simulink model "FOC_Motor_Control"  (R2020b)
settings: Solver=FixedStepAuto  StartTime=0.0  StopTime=10.0  FixedStep=Fixed_Step_Size  RelTol=1e-3
values from neighbouring files (symbols this model uses):
  atan_table = -1.5690511 -1.5690503 -1.5690495 -1.5690485 -1.5690477 -1.5690469 -1.569046 -1.5690452 -1.5690442 -1.5690434 -1.5690426 -1.5690417 -1.5690409 -1.5690399 -1.5690391 -1.5690383 -1.5690374 -1.5690365 -1.5690356 -1.5690348 -1.5690339 -1.569033 -1.5690322 -1.5690314 -1.5690304 -1.5690296 -1.5690287 -1.5690278 -1.5690269 -1.5690261 -1.5690252 -1.5690243 -1.5690234 -1.5690225 -1.5690217 -1.5690207 -1.569    [Motor_Control_Data.sldd]
  Cosine_table = 1.0 0.99999529 0.99999058 0.99998587 0.99998116 0.99996704 0.99995291 0.99993885 0.99992472 0.99990118 0.99987763 0.99985409 0.9998306 0.99979764 0.99976468 0.99973178 0.99969882 0.99965644 0.99961412 0.99957174 0.99952942 0.99947762 0.99942589 0.99937415 0.99932235 0.9992612 0.99920005 0.99913889 0.99907768 0.99900717 0.99893659 0.99886602 0.99879545 0.99871546 0.99863547 0.99855554 0.99847555 0.    [Motor_Control_Data.sldd]
  Dead_Com_Enable = 1.0    [Motor_Control_Data.sldd]
  Dead_Time = 2.5E-6    [Motor_Control_Data.sldd]
  Flux = 0.1125    [Motor_Control_Data.sldd]
  ID_Ki = 48.0    [Motor_Control_Data.sldd]
  ID_Kp = 0.84    [Motor_Control_Data.sldd]
  IQ_Ki = 48.0    [Motor_Control_Data.sldd]
  IQ_Kp = 1.869    [Motor_Control_Data.sldd]
  Ld = 0.00014    [Motor_Control_Data.sldd]
  Lq = 0.0003115    [Motor_Control_Data.sldd]
  Pole_Pairs = 4.0    [Motor_Control_Data.sldd]
  PWM_Frequency = 10000.0    [Motor_Control_Data.sldd]
  Sine_table = 0.0 0.0015339879 0.0030679768 0.0046019657 0.0061359555 0.0076698866 0.0092038177 0.010737749 0.012271681 0.013805497 0.015339312 0.016873131 0.018406944 0.019940587 0.021474229 0.023007872 0.024541514 0.026074925 0.027608337 0.029141748 0.03067516 0.032208283 0.033741407 0.035274528 0.036807653 0.038340431 0.039873205 0.04140598 0.042938754 0.04447113 0.046003502 0.047535874 0.049068246 0.0506001    [Motor_Control_Data.sldd]
  Speed_Ki = 10.809    [Motor_Control_Data.sldd]
  Speed_Kp = 0.08    [Motor_Control_Data.sldd]
  Speed_PI_OutputMax = 700.0    [Motor_Control_Data.sldd]
  Speed_PI_OutputMin = -700.0    [Motor_Control_Data.sldd]
  SpeedFilter_Fn = 0.2    [Motor_Control_Data.sldd]
  TorqueMode = 0.0    [Motor_Control_Data.sldd]
undefined symbols (not defined in the file or in its folder): DiscIntNeverNeededParam, inverter, LADRC_b0, LADRC_Omega_c, SVPWM
libraries: simulink x6
(part 1 of 2)
settings Model: DataDictionary=Motor_Control_Data.sldd  Creator=Administrator  LastModifiedBy=Administrator
settings OptimizationCC: DefaultParameterBehavior=Inlined  UseDivisionForNetSlopeComputation=on  GainParamInheritBuiltInType=on  UseFloatMulNetSlope=on  InlineInvariantSignals=on  PassReuseOutputArgsAs=Individual arguments  ZeroExternalMemoryAtStartup=off  ZeroInternalMemoryAtStartup=off  NoFixptDivByZeroProtection=on  EfficientFloat2IntCast=on  LifeSpan=1  OptimizeBlockOrder=speed  DifferentSizesBufferReuse=on  EfficientTunableParamExpr=on
settings DebuggingCC: ParameterTunabilityLossMsg=error
settings HardwareCC: ProdBitPerPointer=32  ProdBitPerSizeT=32  ProdBitPerPtrDiffT=32  ProdLargestAtomicInteger=Long  ProdLargestAtomicFloat=Double  ProdEndianess=BigEndian  ProdWordSize=32  ProdLongLongMode=on  ProdHWDeviceType=Freescale->32-bit PowerPC
settings ModelReferenceCC: ModelReferenceNumInstancesAllowed=Single
settings SFSimCC: MATLABDynamicMemAlloc=off
settings RTWCC: Description=Embedded Coder  SystemTargetFile=ert.tlc  GenCodeOnly=on  TemplateMakefile=ert_default_tmf  GenerateReport=on  BuildConfiguration=Faster Runs  LaunchReport=on
settings CodeAppCC: ForceParamTrailComments=on  IgnoreCustomStorageClasses=off  OperatorAnnotations=on  SimulinkDataObjDesc=on  SFDataObjDesc=on  CustomSymbolStrGlobalVar=rt$N$M  CustomSymbolStrType=$N$M  CustomSymbolStrFcn=$N$M$F  CustomSymbolStrMacro=$N$M  InsertBlockDesc=on
settings ERTTargetCC: TargetLangStandard=C99 (ISO)  GenerateSampleERTMain=on  IncludeMdlTerminateFcn=off  CombineSignalStateStructs=on  SupportComplex=off  SupportNonInlinedSFcns=on  InlinedParameterPlacement=NonHierarchical  ERTCustomFileTemplate=example_file_process.tlc

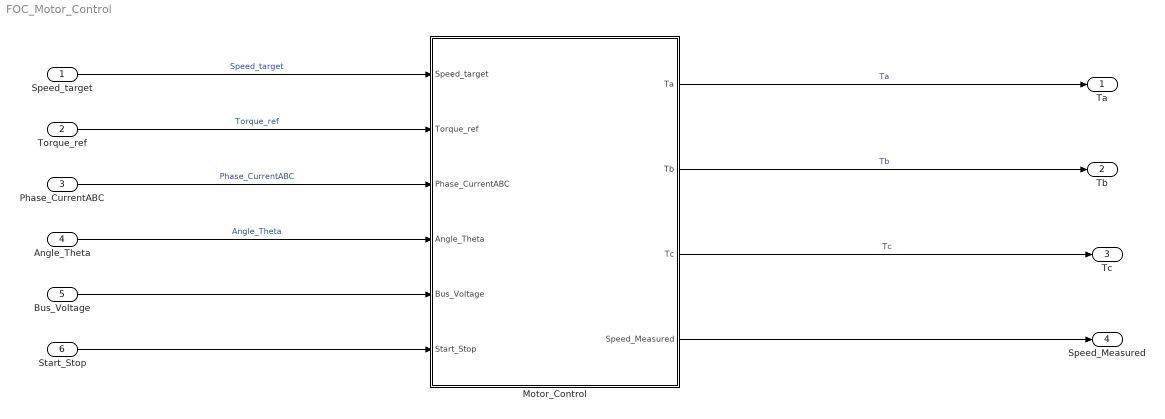
== system FOC_Motor_Control ==
  Speed_target : Inport
  Torque_ref : Inport  Port=2  OutMin=0  OutMax=2*pi  OutDataTypeStr=single
  Phase_CurrentABC : Inport  Port=3  OutDataTypeStr=single  PortDimensions=3
  Angle_Theta : Inport  Port=4  OutMin=0  OutMax=2*pi
  Bus_Voltage : Inport  Port=5
  Start_Stop : Inport  Port=6
  Motor_Control : Subsystem  TreatAsAtomicUnit=on
  Ta : Outport
  Tb : Outport  Port=2
  Tc : Outport  Port=3
  Speed_Measured : Outport  Port=4
  wires:
  Speed_target/1 -> Motor_Control/1(Speed_target)  "Speed_target"
  Motor_Control/1(Ta) -> Ta/1  "Ta"
  Motor_Control/3(Tc) -> Tc/1  "Tc"
  Motor_Control/2(Tb) -> Tb/1  "Tb"
  Phase_CurrentABC/1 -> Motor_Control/3(Phase_CurrentABC)  "Phase_CurrentABC"
  Angle_Theta/1 -> Motor_Control/4(Angle_Theta)  "Angle_Theta"
  Torque_ref/1 -> Motor_Control/2(Torque_ref)  "Torque_ref"
  Bus_Voltage/1 -> Motor_Control/5(Bus_Voltage)
  Start_Stop/1 -> Motor_Control/6(Start_Stop)
  Motor_Control/4(Speed_Measured) -> Speed_Measured/1

== system FOC_Motor_Control/Motor_Control ==
  Speed_target : Inport
  Torque_ref : Inport  Port=2  OutMin=0  OutMax=2*pi
  Phase_CurrentABC : Inport  Port=3  PortDimensions=3
  Angle_Theta : Inport  Port=4  OutMin=0  OutMax=2*pi
  Bus_Voltage : Inport  Port=5
  Start_Stop : Inport  Port=6
  Motor_Control_Function : Subsystem
  Ta : Outport
  Tb : Outport  Port=2
  Tc : Outport  Port=3
  Speed_Measured : Outport  Port=4
  wires:
  Motor_Control_Function/2(Tb) -> Tb/1
  Motor_Control_Function/3(Tc) -> Tc/1
  Motor_Control_Function/1(Ta) -> Ta/1
  Speed_target/1 -> Motor_Control_Function/1(Speed_target)  "Speed_target"
  Phase_CurrentABC/1 -> Motor_Control_Function/2(Phase_CurrentABC)  "Phase_CurrentABC"
  Angle_Theta/1 -> Motor_Control_Function/3(Angle_Theta)  "Angle_Theta"
  Start_Stop/1 -> Motor_Control_Function/5(Start_Stop)
  Bus_Voltage/1 -> Motor_Control_Function/4(Bus_voltage)
  Torque_ref/1 -> Motor_Control_Function/6(Torque_ref)
  Motor_Control_Function/5(Speed_Measured) -> Speed_Measured/1

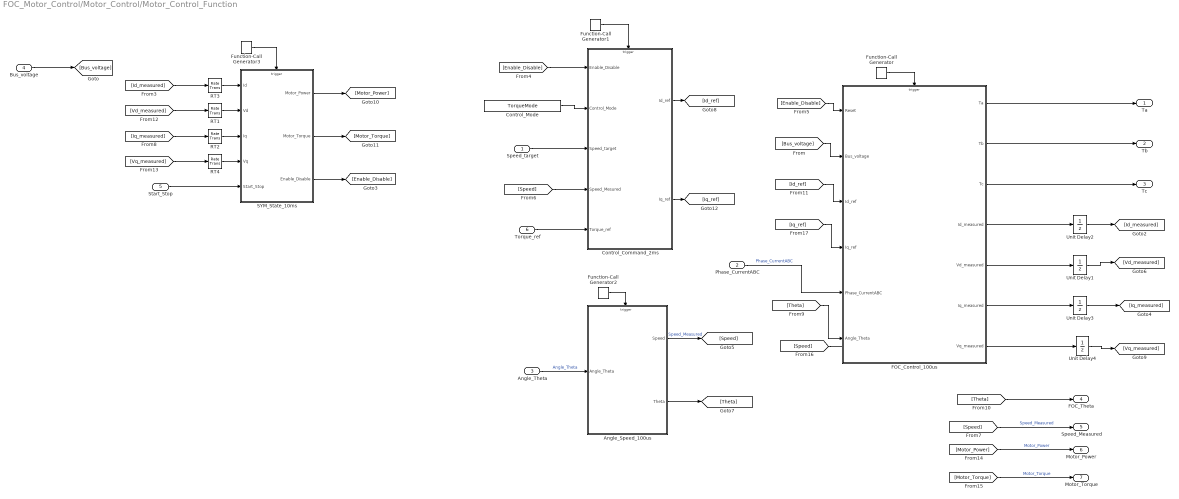
== system FOC_Motor_Control/Motor_Control/Motor_Control_Function ==
  Speed_target : Inport
  Phase_CurrentABC : Inport  Port=2  PortDimensions=3
  Angle_Theta : Inport  Port=3  OutMin=0  OutMax=2*pi
  Bus_voltage : Inport  Port=4
  Start_Stop : Inport  Port=5
  Torque_ref : Inport  Port=6  OutMin=0  OutMax=2*pi
  Angle_Speed_100us : Subsystem
      settings: RTWSystemCode=Nonreusable function  RTWFcnNameOpts=Use subsystem name  RTWFileNameOpts=Use subsystem name
  Control_Command_2ms : Subsystem  TreatAsAtomicUnit=on
      settings: RTWSystemCode=Nonreusable function  RTWFcnNameOpts=Use subsystem name  RTWFileNameOpts=Use subsystem name  FunctionInterfaceSpec=Allow arguments (Optimized)
  Control_Mode : Constant  Value=TorqueMode
  FOC_Control_100us : Subsystem  TreatAsAtomicUnit=on
      settings: RTWSystemCode=Nonreusable function  RTWFcnNameOpts=Use subsystem name  RTWFileNameOpts=Use subsystem name  FunctionInterfaceSpec=Allow arguments (Optimized)
  Function-Call Generator : simulink/Ports & Subsystems/Function-Call Generator  sample_time=1/PWM_Frequency  numberOfIterations=1  DisallowWideOutput=off
  Function-Call Generator1 : simulink/Ports & Subsystems/Function-Call Generator  sample_time=Task_2ms  numberOfIterations=1  DisallowWideOutput=off
  Function-Call Generator2 : simulink/Ports & Subsystems/Function-Call Generator  sample_time=1/PWM_Frequency  numberOfIterations=1  DisallowWideOutput=off
  Function-Call Generator3 : simulink/Ports & Subsystems/Function-Call Generator  sample_time=Task_10ms  numberOfIterations=1  DisallowWideOutput=off
  RT{1..4} (4 alike) : RateTransition  Integrity=off
  SYM_State_10ms : Subsystem
      settings: RTWSystemCode=Nonreusable function  RTWFcnNameOpts=Use subsystem name  RTWFileNameOpts=Use subsystem name
  Unit Delay{1..4} (4 alike) : UnitDelay  SampleTime=-1  HasFrameUpgradeWarning=on
  Ta : Outport
  Tb : Outport  Port=2
  Tc : Outport  Port=3
  FOC_Theta : Outport  Port=4
  Speed_Measured : Outport  Port=5
  Motor_Power : Outport  Port=6
  Motor_Torque : Outport  Port=7
  wires:
  Function-Call Generator1/1 -> Control_Command_2ms/Trigger
  Control_Mode/1 -> Control_Command_2ms/2(Control_Mode)
  Angle_Theta/1 -> Angle_Speed_100us/1(Angle_Theta)  "Angle_Theta"
  Function-Call Generator/1 -> FOC_Control_100us/Trigger
  Phase_CurrentABC/1 -> FOC_Control_100us/5(Phase_CurrentABC)  "Phase_CurrentABC"
  FOC_Control_100us/3(Tc) -> Tc/1
  Speed_target/1 -> Control_Command_2ms/3(Speed_target)
  FOC_Control_100us/2(Tb) -> Tb/1
  FOC_Control_100us/1(Ta) -> Ta/1
  Function-Call Generator2/1 -> Angle_Speed_100us/Trigger
  Function-Call Generator3/1 -> SYM_State_10ms/Trigger
  SYM_State_10ms/3(Enable_Disable) -> [Enable_Disable]
  [Enable_Disable] -> Control_Command_2ms/1(Enable_Disable)
  [Enable_Disable] -> FOC_Control_100us/1(Reset)
  Angle_Speed_100us/1(Speed) -> [Speed]  "Speed_Measured"
  [Speed] -> Speed_Measured/1  "Speed_Measured"
  Angle_Speed_100us/2(Theta) -> [Theta]
  [Theta] -> FOC_Control_100us/6(Angle_Theta)
  [Theta] -> FOC_Theta/1
  Control_Command_2ms/1(Id_ref) -> [Id_ref]
  [Id_ref] -> FOC_Control_100us/3(Id_ref)
  Start_Stop/1 -> SYM_State_10ms/5(Start_Stop)
  Bus_voltage/1 -> [Bus_voltage]
  FOC_Control_100us/6(Iq_measured) -> Unit Delay3/1
  FOC_Control_100us/7(Vq_measured) -> Unit Delay4/1
  FOC_Control_100us/4(Id_measured) -> Unit Delay2/1
  FOC_Control_100us/5(Vd_measured) -> Unit Delay1/1
  Unit Delay2/1 -> [Id_measured]
  Unit Delay1/1 -> [Vd_measured]
  Unit Delay3/1 -> [Iq_measured]
  Unit Delay4/1 -> [Vq_measured]
  [Iq_measured] -> RT2/1
  [Id_measured] -> RT3/1
  [Vd_measured] -> RT1/1
  [Vq_measured] -> RT4/1
  SYM_State_10ms/1(Motor_Power) -> [Motor_Power]
  [Motor_Power] -> Motor_Power/1  "Motor_Power"
  RT3/1 -> SYM_State_10ms/1(Id)
  RT1/1 -> SYM_State_10ms/2(Vd)
  RT2/1 -> SYM_State_10ms/3(Iq)
  RT4/1 -> SYM_State_10ms/4(Vq)
  [Bus_voltage] -> FOC_Control_100us/2(Bus_voltage)
  SYM_State_10ms/2(Motor_Torque) -> [Motor_Torque]
  [Motor_Torque] -> Motor_Torque/1  "Motor_Torque"
  Torque_ref/1 -> Control_Command_2ms/5(Torque_ref)
  [Speed] -> ?
  [Speed] -> Control_Command_2ms/4(Speed_Mesured)
  Control_Command_2ms/2(Iq_ref) -> [Iq_ref]
  [Iq_ref] -> FOC_Control_100us/4(Iq_ref)

== system FOC_Motor_Control/Motor_Control/Motor_Control_Function/Angle_Speed_100us ==
  Angle_Theta : Inport  OutMin=0  OutMax=2*pi
  Trigger : TriggerPort  TriggerType=function-call  VariantControl=Variant  SampleTimeType=periodic  SampleTime=-1  PortDimensions=1
  Speed_Resolver : Subsystem  TreatAsAtomicUnit=on
      settings: RTWSystemCode=Nonreusable function  RTWFcnNameOpts=Use subsystem name
  Speed : Outport
  Theta : Outport  Port=2
  wires:
  Speed_Resolver/1(Speed_out) -> Speed/1
  Speed_Resolver/2(Dir_Angle) -> Theta/1
  Angle_Theta/1 -> Speed_Resolver/1(Theta)  "Angle_Theta"

== system FOC_Motor_Control/Motor_Control/Motor_Control_Function/Control_Command_2ms ==
  Enable_Disable : Inport
  Control_Mode : Inport  Port=2
  Speed_target : Inport  Port=3
  Speed_Mesured : Inport  Port=4  OutMin=0  OutMax=2*pi
  Torque_ref : Inport  Port=5  OutMin=0  OutMax=2*pi
  Trigger : TriggerPort  TriggerType=function-call  VariantControl=Variant  SampleTimeType=periodic  SampleTime=-1  PortDimensions=1
  Constant : Constant  Value=0  OutDataTypeStr=single
  Control_Command_2ms : Subsystem  TreatAsAtomicUnit=on
      settings: RTWSystemCode=Nonreusable function  RTWFcnNameOpts=Use subsystem name  RTWFileNameOpts=Use subsystem name  FunctionInterfaceSpec=Allow arguments (Optimized)
  Id_ref : Outport
  Iq_ref : Outport  Port=2
  wires:
  Control_Mode/1 -> Control_Command_2ms/2(Control_Mode)
  Speed_target/1 -> Control_Command_2ms/3(Speed_target)
  Speed_Mesured/1 -> Control_Command_2ms/4(Speed_Mesured)
  Enable_Disable/1 -> Control_Command_2ms/1(Reset)
  Torque_ref/1 -> Control_Command_2ms/5(Torque_ref)
  Control_Command_2ms/1(Te_ref) -> Iq_ref/1  "Iq_ref"
  Constant/1 -> Id_ref/1  "Id_ref"

== system FOC_Motor_Control/Motor_Control/Motor_Control_Function/FOC_Control_100us ==
  Reset : Inport
  Bus_voltage : Inport  Port=2
  Id_ref : Inport  Port=3
  Iq_ref : Inport  Port=4
  Phase_CurrentABC : Inport  Port=5  PortDimensions=3
  Angle_Theta : Inport  Port=6  OutMin=0  OutMax=2*pi
  Trigger : TriggerPort  TriggerType=function-call  VariantControl=Variant  SampleTimeType=periodic  SampleTime=-1  PortDimensions=1
  FOC : Subsystem  TreatAsAtomicUnit=on
      settings: RTWSystemCode=Nonreusable function  RTWFcnNameOpts=Use subsystem name
  Ta : Outport
  Tb : Outport  Port=2
  Tc : Outport  Port=3
  Id_measured : Outport  Port=4
  Vd_measured : Outport  Port=5
  Iq_measured : Outport  Port=6
  Vq_measured : Outport  Port=7
  wires:
  FOC/1(Ta) -> Ta/1  "Ta"
  FOC/2(Tb) -> Tb/1  "Tb"
  FOC/3(Tc) -> Tc/1  "Tc"
  Angle_Theta/1 -> FOC/5(Angle_Theta)  "Angle_Theta"
  Phase_CurrentABC/1 -> FOC/6(Phase_CurrentABC)  "Phase_CurrentABC"
  Reset/1 -> FOC/1(Reset)
  FOC/6(Iq_measured) -> Iq_measured/1
  FOC/7(Vq_measured) -> Vq_measured/1
  FOC/4(Id_measured) -> Id_measured/1
  FOC/5(Vd_measured) -> Vd_measured/1
  Bus_voltage/1 -> FOC/2(Bus_voltage)
  Id_ref/1 -> FOC/3(Id_target)  "Id_ref"
  Iq_ref/1 -> FOC/4(Iq_target)  "Iq_ref"

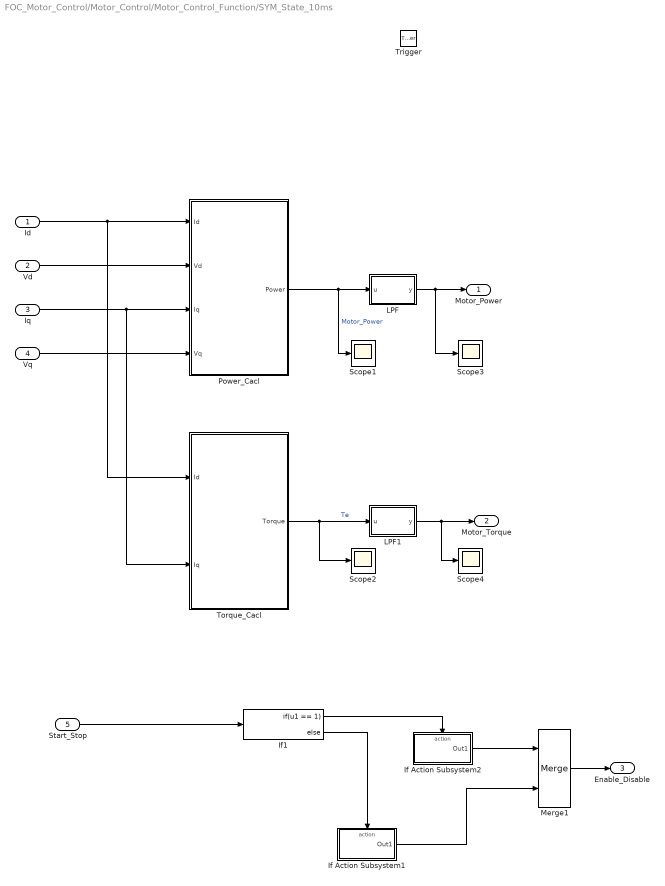
== system FOC_Motor_Control/Motor_Control/Motor_Control_Function/SYM_State_10ms ==
  Id : Inport
  Vd : Inport  Port=2
  Iq : Inport  Port=3
  Vq : Inport  Port=4
  Start_Stop : Inport  Port=5  OutDataTypeStr=uint8
  Trigger : TriggerPort  TriggerType=function-call  VariantControl=Variant  SampleTimeType=periodic  SampleTime=-1  PortDimensions=1
  If Action Subsystem1 : Subsystem  TreatAsAtomicUnit=on
  If Action Subsystem2 : Subsystem  TreatAsAtomicUnit=on
  If1 : If  IfExpression=u1 == 1
  LPF : Subsystem
  LPF1 : Subsystem
  Merge1 : Merge
  Power_Cacl : Subsystem
  Scope{1..4} (4 alike) : Scope
  Torque_Cacl : Subsystem
  Motor_Power : Outport
  Motor_Torque : Outport  Port=2
  Enable_Disable : Outport  Port=3
  wires:
  Iq/1 -> Torque_Cacl/2(Iq), Power_Cacl/3(Iq)
  Vq/1 -> Power_Cacl/4(Vq)
  Power_Cacl/1(Power) -> LPF/1(u), Scope1/1  "Motor_Power"
  Vd/1 -> Power_Cacl/2(Vd)
  Id/1 -> Torque_Cacl/1(Id), Power_Cacl/1(Id)
  LPF/1(y) -> Scope3/1, Motor_Power/1
  Torque_Cacl/1(Torque) -> LPF1/1(u), Scope2/1  "Te"
  LPF1/1(y) -> Motor_Torque/1, Scope4/1
  Start_Stop/1 -> If1/1
  If1/2 -> If Action Subsystem1/Action
  If1/1 -> If Action Subsystem2/Action
  If Action Subsystem2/1(Out1) -> Merge1/1
  If Action Subsystem1/1(Out1) -> Merge1/2
  Merge1/1 -> Enable_Disable/1

== system FOC_Motor_Control/Motor_Control/Motor_Control_Function/Angle_Speed_100us/Speed_Resolver ==
  Theta : Inport
  DT2 : DataTypeConversion  OutDataTypeStr=single
  Speed_cacl : Subsystem  TreatAsAtomicUnit=on
      settings: RTWSystemCode=Nonreusable function  RTWFcnNameOpts=Use subsystem name
  Speed_out : Outport
  Dir_Angle : Outport  Port=2
  wires:
  Theta/1 -> DT2/1, Speed_cacl/1(position)
  Speed_cacl/1(Speed_RPM) -> Speed_out/1  "Speed_Measured"
  DT2/1 -> Dir_Angle/1  "Direct_Angle"

== system FOC_Motor_Control/Motor_Control/Motor_Control_Function/Control_Command_2ms/Control_Command_2ms ==
  Reset : Inport
  Control_Mode : Inport  Port=2
  Speed_target : Inport  Port=3
  Speed_Mesured : Inport  Port=4  OutMin=0  OutMax=2*pi
  Torque_ref : Inport  Port=5  OutMin=0  OutMax=2*pi
  Merge : Merge
  Speed_PI : Subsystem  TreatAsAtomicUnit=on  SystemSampleTime=inverter.Ts
      settings: RTWSystemCode=Nonreusable function
  Switch Case : SwitchCase  CaseConditions={0,1}
  Switch Case Action Subsystem : Subsystem  TreatAsAtomicUnit=on
      settings: RTWSystemCode=Nonreusable function
  Te_ref : Outport
  wires:
  Switch Case Action Subsystem/1(Iq_out) -> Merge/2
  Torque_ref/1 -> Switch Case Action Subsystem/1(Iq_in)
  Switch Case/3 -> [default]
  [Torque_Mode] -> Switch Case Action Subsystem/Action
  Switch Case/2 -> [Torque_Mode]
  Switch Case/1 -> [Speed_Mode]
  Control_Mode/1 -> Switch Case/1
  [Speed_Mode] -> Speed_PI/Action
  Speed_PI/1(Iq_ref) -> Merge/1  "Iq_ref"
  Merge/1 -> Te_ref/1
  Speed_target/1 -> Speed_PI/1(Speed_Command)
  Reset/1 -> Speed_PI/3(Reset)
  Speed_Mesured/1 -> Speed_PI/2(Speed_Measured)

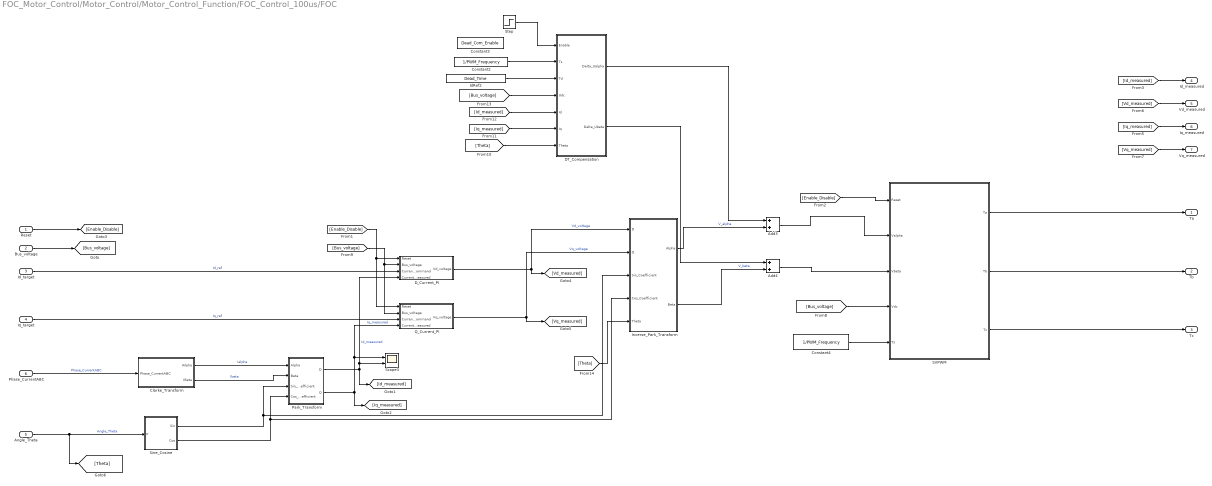
== system FOC_Motor_Control/Motor_Control/Motor_Control_Function/FOC_Control_100us/FOC ==
  Reset : Inport
  Bus_voltage : Inport  Port=2
  Id_target : Inport  Port=3
  Iq_target : Inport  Port=4
  Angle_Theta : Inport  Port=5  OutMin=0  OutMax=2*pi
  Phase_CurrentABC : Inport  Port=6  PortDimensions=3
  Add3 : Sum  OutDataTypeStr=single
  Add4 : Sum  OutDataTypeStr=single
  Clarke_Transform : Subsystem  TreatAsAtomicUnit=on
      settings: RTWSystemCode=Nonreusable function  RTWFcnNameOpts=Use subsystem name
  Constant2 : Constant  Value=1/PWM_Frequency  OutDataTypeStr=single
  Constant3 : Constant  Value=Dead_Com_Enable  OutDataTypeStr=single
  Constant4 : Constant  Value=1/PWM_Frequency  OutDataTypeStr=single
  DT_Compensation : Subsystem  TreatAsAtomicUnit=on
      settings: RTWSystemCode=Nonreusable function  RTWFcnNameOpts=Use subsystem name
  D_Current_PI : Subsystem  TreatAsAtomicUnit=on
      settings: RTWSystemCode=Nonreusable function  RTWFcnNameOpts=Use subsystem name
  IdRef2 : Constant  Value=Dead_Time  OutDataTypeStr=single
  Inverse_Park_Transform : Subsystem  TreatAsAtomicUnit=on
      settings: RTWSystemCode=Nonreusable function  RTWFcnNameOpts=Use subsystem name
      mask Display:
      | port_label('input',1,'D')
      | port_label('input',2,'Q')
      | port_label('input',3,'Sin')
      | port_label('input',4,'Cos')
      | port_label('output',1,'\alpha','texmode', 'on')
      | port_label('output',2,'\beta','texmode', 'on')
  Park_Transform : Subsystem  TreatAsAtomicUnit=on
      settings: RTWSystemCode=Nonreusable function  RTWFcnNameOpts=Use subsystem name
      mask Display:
      | port_label('input',1,'\alpha','texmode', 'on')
      | port_label('input',2,'\beta','texmode', 'on')
      | port_label('input',3,'Sin')
      | port_label('input',4,'Cos')
      | port_label('output',1,'D')
      | port_label('output',2,'Q')
  Q_Current_PI : Subsystem  TreatAsAtomicUnit=on
      settings: RTWSystemCode=Nonreusable function  RTWFcnNameOpts=Use subsystem name
  SVPWM : Subsystem  AncestorBlock=SVPWM/SVPWM  TreatAsAtomicUnit=on  RTWFcnName=SVPWM  RTWFileName=SVPWM
      settings: RTWSystemCode=Nonreusable function  RTWFcnNameOpts=Use subsystem name
      mask Display:
      | plot([0.000 0.020 0.041 0.061 0.082 0.102 0.122 0.143 0.163 0.184 0.204 0.224 0.245 0.265 0.286 0.306 0.327 0.347 0.367 0.388 0.408 0.429 0.449 0.469 0.490 0.510 0.531 0.551 0.571 0.592 0.612 0.633 0.653 0.673 0.694 0.714 0.735 0.755 0.776 0.796 0.816 0.837 0.857 0.878 0.898 0.918 0.939 0.959 0.980 1.000 ], ...
      |      [0.500 0.586 0.671 0.753 0.831 0.858 0.875 0.885 0.890 0.887 0.879 0.864 0.844 0.855 0.872 0.884 0.889 0.888 0.881 0.867 0.847 0.793 0.713 0.629 0.543 0.457 0.371 0.287 0.207 0.153 0.133 0.119 0.112 0.111 0.116 0.128 0.145 0.156 0.136 0.121 0.113 0.110 0.115 0.125 0.142 0.169 0.247 0.329 0.414 0.500 ])
  Scope3 : Scope  NumInputPorts=2
  Sine_Cosine : Subsystem  TreatAsAtomicUnit=on
      settings: RTWSystemCode=Nonreusable function  RTWFcnNameOpts=Use subsystem name
  Step : Step  Time=0.3
  Ta : Outport
  Tb : Outport  Port=2
  Tc : Outport  Port=3
  Id_measured : Outport  Port=4
  Vd_measured : Outport  Port=5
  Iq_measured : Outport  Port=6
  Vq_measured : Outport  Port=7
  wires:
  Park_Transform/1(D) -> Scope3/2, D_Current_PI/4(Current_Measured), [Id_measured]  "Id_measured"
  Constant4/1 -> SVPWM/5(Ts)
  Park_Transform/2(Q) -> Q_Current_PI/4(Current_Measured), Scope3/1, [Iq_measured]  "Iq_measured"
  Sine_Cosine/2(Cos) -> Park_Transform/4(Cos_Coefficient), Inverse_Park_Transform/4(Cos_Coefficient)
  Sine_Cosine/1(Sin) -> Park_Transform/3(Sin_Coefficient), Inverse_Park_Transform/3(Sin_Coefficient)
  [Bus_voltage] -> SVPWM/4(Vdc)
  D_Current_PI/1(Vd_voltage) -> [Vd_measured], Inverse_Park_Transform/1(D)  "Vd_voltage"
  Q_Current_PI/1(Vq_voltage) -> [Vq_measured], Inverse_Park_Transform/2(Q)  "Vq_voltage"
  Clarke_Transform/2(IBeta) -> Park_Transform/2(Beta)  "Ibeta"
  Clarke_Transform/1(IAlpha) -> Park_Transform/1(Alpha)  "Ialpha"
  Iq_target/1 -> Q_Current_PI/3(Current_Command)  "Iq_ref"
  Phase_CurrentABC/1 -> Clarke_Transform/1(Phase_CurrentABC)  "Phase_CurrentABC"
  Angle_Theta/1 -> [Theta], Sine_Cosine/1(P)  "Angle_Theta"
  Id_target/1 -> D_Current_PI/3(Current_Command)  "Id_ref"
  Reset/1 -> [Enable_Disable]
  [Enable_Disable] -> D_Current_PI/1(Reset), Q_Current_PI/1(Reset)
  [Enable_Disable] -> SVPWM/1(Reset)
  [Iq_measured] -> Iq_measured/1
  [Id_measured] -> Id_measured/1
  [Vd_measured] -> Vd_measured/1
  [Vq_measured] -> Vq_measured/1
  Bus_voltage/1 -> [Bus_voltage]
  [Bus_voltage] -> D_Current_PI/2(Bus_voltage), Q_Current_PI/2(Bus_voltage)
  SVPWM/1(Ta) -> Ta/1
  SVPWM/2(Tb) -> Tb/1
  SVPWM/3(Tc) -> Tc/1
  [Bus_voltage] -> DT_Compensation/4(Udc)
  Constant2/1 -> DT_Compensation/2(Ts)
  IdRef2/1 -> DT_Compensation/3(Td)
  Inverse_Park_Transform/1(Alpha) -> Add3/2  "V_alpha"
  Add3/1 -> SVPWM/2(Valpha)
  Inverse_Park_Transform/2(Beta) -> Add4/2  "V_beta"
  Add4/1 -> SVPWM/3(Vbeta)
  [Id_measured] -> DT_Compensation/5(Id)
  [Iq_measured] -> DT_Compensation/6(Iq)
  [Theta] -> DT_Compensation/7(Theta)
  DT_Compensation/2(Delta_Ubeta) -> Add4/1
  DT_Compensation/1(Delta_Ualpha) -> Add3/1
  [Theta] -> Inverse_Park_Transform/5(Theta)
  Step/1 -> DT_Compensation/1(Enable)

== system FOC_Motor_Control/Motor_Control/Motor_Control_Function/SYM_State_10ms/If Action Subsystem1 ==
  Action Port : ActionPort  ActionPortLabel=else
  Disable : Constant  OutDataTypeStr=uint8
  Out1 : Outport
  wires:
  Disable/1 -> Out1/1

== system FOC_Motor_Control/Motor_Control/Motor_Control_Function/SYM_State_10ms/If Action Subsystem2 ==
  Action Port : ActionPort  ActionPortLabel=if(u1 == 1)
  enable : Constant  Value=0  OutDataTypeStr=uint8
  Out1 : Outport
  wires:
  enable/1 -> Out1/1

== system FOC_Motor_Control/Motor_Control/Motor_Control_Function/SYM_State_10ms/LPF ==
  u : Inport
  Add : Sum  Inputs=+-
  Add1 : Sum
  Constant1 : Constant  Value=0.005  OutDataTypeStr=single
  Divide1 : Product  Inputs=**
  Unit Delay : UnitDelay  SampleTime=-1  HasFrameUpgradeWarning=on
  y : Outport
  wires:
  Constant1/1 -> Divide1/1
  u/1 -> Add/1
  Add/1 -> Divide1/2
  Divide1/1 -> Add1/1
  Unit Delay/1 -> Add/2, Add1/2
  Add1/1 -> Unit Delay/1, y/1

== system FOC_Motor_Control/Motor_Control/Motor_Control_Function/SYM_State_10ms/LPF1 ==
  u : Inport
  Add : Sum  Inputs=+-
  Add1 : Sum
  Constant1 : Constant  Value=0.005  OutDataTypeStr=single
  Divide1 : Product  Inputs=**
  Unit Delay : UnitDelay  SampleTime=-1  HasFrameUpgradeWarning=on
  y : Outport
  wires:
  Constant1/1 -> Divide1/1
  u/1 -> Add/1
  Add/1 -> Divide1/2
  Divide1/1 -> Add1/1
  Unit Delay/1 -> Add/2, Add1/2
  Add1/1 -> Unit Delay/1, y/1

== system FOC_Motor_Control/Motor_Control/Motor_Control_Function/SYM_State_10ms/Power_Cacl ==
  Id : Inport
  Vd : Inport  Port=2
  Iq : Inport  Port=3
  Vq : Inport  Port=4
  Add : Sum
  Product : Product
  Product1 : Product
  Power : Outport
  wires:
  Id/1 -> Product/1
  Vd/1 -> Product/2
  Iq/1 -> Product1/1
  Vq/1 -> Product1/2
  Product/1 -> Add/1
  Product1/1 -> Add/2
  Add/1 -> Power/1

== system FOC_Motor_Control/Motor_Control/Motor_Control_Function/SYM_State_10ms/Torque_Cacl ==
  Id : Inport
  Iq : Inport  Port=2
  Constant : Constant  Value=3/2  OutDataTypeStr=single
  Constant1 : Constant  Value=Pole_Pairs  OutDataTypeStr=single
  Constant2 : Constant  Value=Flux  OutDataTypeStr=single
  Constant3 : Constant  Value=Ld  OutDataTypeStr=single
  Constant4 : Constant  Value=Lq  OutDataTypeStr=single
  Product{,1..4} (5 alike) : Product
  Subtract : Sum
  Subtract1 : Sum  Inputs=+-
  Torque : Outport
  wires:
  Constant1/1 -> Product/1
  Constant/1 -> Product/2
  Constant2/1 -> Product1/1
  Iq/1 -> Product1/2, Product3/1
  Product1/1 -> Subtract/1
  Constant3/1 -> Subtract1/1
  Constant4/1 -> Subtract1/2
  Subtract1/1 -> Product2/1
  Id/1 -> Product2/2
  Product2/1 -> Product3/2
  Product3/1 -> Subtract/2
  Product/1 -> Product4/1
  Subtract/1 -> Product4/2
  Product4/1 -> Torque/1

== system FOC_Motor_Control/Motor_Control/Motor_Control_Function/Angle_Speed_100us/Speed_Resolver/Speed_cacl ==
  note: Speed_Measured
  position : Inport  OutMin=-4*pi  OutMax=4*pi
      settings: AttributesFormatString="------------------\\nMin =  %<OutMin>\\nMax =  %<OutMax>"
  Constant : Constant  Value=pi/(2^31 -1)/(1/PWM_Frequency)  OutDataTypeStr=single
  Constant1 : Constant  Value=1/Pole_Pairs  OutDataTypeStr=single
  Difference_Wrap : Sum  Inputs=+-  AccumDataTypeStr=int32  OutDataTypeStr=int32
  Difference_to_Single : DataTypeConversion  OutDataTypeStr=single
  Difference_to_Single1 : DataTypeConversion  OutDataTypeStr=int32
  Gain : Gain  Gain=60/(2*pi)
  LPF : Subsystem
  Position_Delay : Delay  DelayLength=1
  Product : Product
  Product1 : Product
  Scale_Input : Gain  Gain=((2^31) - 1)/(4*pi)  ParamDataTypeStr=single  OutDataTypeStr=single
      settings: AttributesFormatString=---------------------------------\n%<Gain>
  Scope : Scope  NumInputPorts=2
  Wrap_To_Pi : Gain  Gain=4  RndMeth=Simplest  OutDataTypeStr=Inherit: Same as input  ParamDataTypeStr=Inherit: Same as input
  Speed_RPM : Outport  VectorParamsAs1DForOutWhenUnconnected=off
  wires:
  position/1 -> Scale_Input/1  "position"
  Difference_to_Single/1 -> Product/2
  Wrap_To_Pi/1 -> Difference_Wrap/1, Position_Delay/1
  Position_Delay/1 -> Difference_Wrap/2
  Scale_Input/1 -> Difference_to_Single1/1
  Difference_Wrap/1 -> Difference_to_Single/1
  Constant/1 -> Product/1
  Constant1/1 -> Product1/1
  Product/1 -> Gain/1  "We"
  Gain/1 -> Product1/2
  Difference_to_Single1/1 -> Wrap_To_Pi/1
  Product1/1 -> Scope/1, LPF/1(u)
  LPF/1(y) -> Scope/2, Speed_RPM/1

== system FOC_Motor_Control/Motor_Control/Motor_Control_Function/Control_Command_2ms/Control_Command_2ms/Speed_PI ==
  Speed_Command : Inport
  Speed_Measured : Inport  Port=2
  Reset : Inport  Port=3
  Action Port : ActionPort  ActionPortLabel=case [ 0 ]:
  SpeedLoop : Subsystem  Commented=on
  Speed_PI : Subsystem
  Iq_ref : Outport  VectorParamsAs1DForOutWhenUnconnected=off
  wires:
  Speed_PI/1(PI_out) -> Iq_ref/1
  Speed_Command/1 -> Speed_PI/1(Ref)
  Reset/1 -> Speed_PI/3(Reset)
  Speed_Measured/1 -> Speed_PI/2(Fdk)

== system FOC_Motor_Control/Motor_Control/Motor_Control_Function/Control_Command_2ms/Control_Command_2ms/Switch Case Action Subsystem ==
  Iq_in : Inport
  Action Port : ActionPort  ActionPortLabel=case [ 1 ]:
  Iq_out : Outport
  wires:
  Iq_in/1 -> Iq_out/1

== system FOC_Motor_Control/Motor_Control/Motor_Control_Function/FOC_Control_100us/FOC/Clarke_Transform ==
  Phase_CurrentABC : Inport  PortDimensions=3
  Clark1 : Subsystem  TreatAsAtomicUnit=on
  Scope : Scope  NumInputPorts=2
  IAlpha : Outport  VectorParamsAs1DForOutWhenUnconnected=off
  IBeta : Outport  Port=2  VectorParamsAs1DForOutWhenUnconnected=off
  wires:
  Clark1/1(Ialpha) -> IAlpha/1, Scope/1
  Clark1/2(Ibeta) -> IBeta/1, Scope/2
  Phase_CurrentABC/1 -> Clark1/1(Iabc)

== system FOC_Motor_Control/Motor_Control/Motor_Control_Function/FOC_Control_100us/FOC/DT_Compensation ==
  Enable : Inport
  Ts : Inport  Port=2
  Td : Inport  Port=3
  Udc : Inport  Port=4
  Id : Inport  Port=5
  Iq : Inport  Port=6
  Theta : Inport  Port=7
  DT_Compensation : Subsystem
  Delta_Ualpha : Outport
  Delta_Ubeta : Outport  Port=2
  wires:
  Enable/1 -> DT_Compensation/Enable
  Td/1 -> DT_Compensation/2(Td)
  Ts/1 -> DT_Compensation/1(Ts)
  Udc/1 -> DT_Compensation/3(Udc)
  Id/1 -> DT_Compensation/4(Id)
  Iq/1 -> DT_Compensation/5(Iq)
  Theta/1 -> DT_Compensation/6(Theta)
  DT_Compensation/2(Delta_Ubeta) -> Delta_Ubeta/1
  DT_Compensation/1(Delta_Ualpha) -> Delta_Ualpha/1

== system FOC_Motor_Control/Motor_Control/Motor_Control_Function/FOC_Control_100us/FOC/D_Current_PI ==
  Reset : Inport
  Bus_voltage : Inport  Port=2
  Current_Command : Inport  Port=3
  Current_Measured : Inport  Port=4
  Add2 : Sum  Inputs=|+-
  ID_Control : Subsystem
  Vd_voltage : Outport  VectorParamsAs1DForOutWhenUnconnected=off
  wires:
  Current_Command/1 -> Add2/1
  Current_Measured/1 -> Add2/2
  Add2/1 -> ID_Control/3(Err)  "currentControlError"
  Reset/1 -> ID_Control/1(Reset)
  Bus_voltage/1 -> ID_Control/2(Bus_voltage)
  ID_Control/1(PI_Out) -> Vd_voltage/1

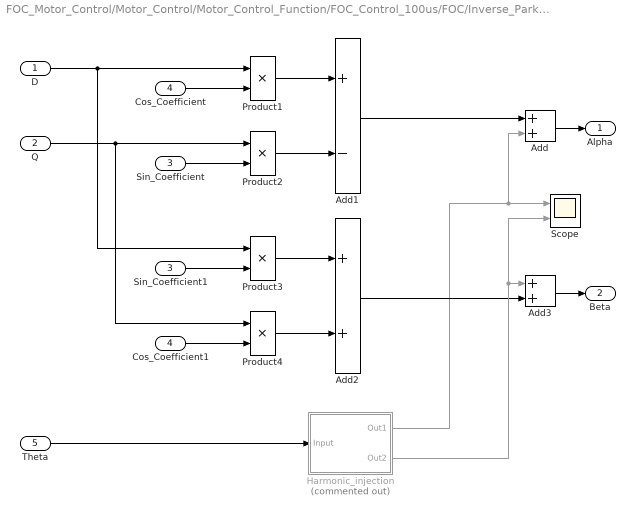
== system FOC_Motor_Control/Motor_Control/Motor_Control_Function/FOC_Control_100us/FOC/Inverse_Park_Transform ==
  D : Inport
  Q : Inport  Port=2
  Sin_Coefficient : Inport  Port=3
  Cos_Coefficient : Inport  Port=4
  Theta : Inport  Port=5
  Add : Sum
  Add1 : Sum  Inputs=+-  OutDataTypeStr=Inherit: Same as first input
  Add2 : Sum  OutDataTypeStr=Inherit: Same as first input
  Add3 : Sum
  Cos_Coefficient1 : InportShadow  Port=4
  Harmonic_injection : Subsystem  Commented=on
  Product{1..4} (4 alike) : Product  RndMeth=Simplest  OutDataTypeStr=Inherit: Same as first input
  Scope : Scope  NumInputPorts=2
  Sin_Coefficient1 : InportShadow  Port=3
  Alpha : Outport  VectorParamsAs1DForOutWhenUnconnected=off
  Beta : Outport  Port=2  VectorParamsAs1DForOutWhenUnconnected=off
  wires:
  Product3/1 -> Add2/1
  Product4/1 -> Add2/2
  Product1/1 -> Add1/1
  Product2/1 -> Add1/2
  Cos_Coefficient1/1 -> Product4/2
  Sin_Coefficient/1 -> Product2/2
  D/1 -> Product3/1, Product1/1
  Q/1 -> Product2/1, Product4/1
  Sin_Coefficient1/1 -> Product3/2
  Cos_Coefficient/1 -> Product1/2
  Add1/1 -> Add/1
  Add/1 -> Alpha/1
  Harmonic_injection/1(Out1) -> Scope/1, Add/2
  Add2/1 -> Add3/2
  Add3/1 -> Beta/1
  Harmonic_injection/2(Out2) -> Scope/2, Add3/1
  Theta/1 -> Harmonic_injection/1(Input)

== system FOC_Motor_Control/Motor_Control/Motor_Control_Function/FOC_Control_100us/FOC/Park_Transform ==
  Alpha : Inport
  Beta : Inport  Port=2
  Sin_Coefficient : Inport  Port=3
  Cos_Coefficient : Inport  Port=4
  Add1 : Sum  OutDataTypeStr=Inherit: Same as first input
  Add2 : Sum  Inputs=-+  OutDataTypeStr=Inherit: Same as first input
  Alpha1 : InportShadow
  Beta1 : InportShadow  Port=2
  Cos_Coefficient1 : InportShadow  Port=4
  Produc3t : Product  RndMeth=Simplest  OutDataTypeStr=Inherit: Same as first input
  Product1 : Product  RndMeth=Simplest  OutDataTypeStr=Inherit: Same as first input
  Product2 : Product  RndMeth=Simplest  OutDataTypeStr=Inherit: Same as first input
  Product4 : Product  RndMeth=Simplest  OutDataTypeStr=Inherit: Same as first input
  Sin_Coefficient1 : InportShadow  Port=3
  D : Outport  VectorParamsAs1DForOutWhenUnconnected=off
  Q : Outport  Port=2  VectorParamsAs1DForOutWhenUnconnected=off
  wires:
  Produc3t/1 -> Add2/1
  Product4/1 -> Add2/2
  Product1/1 -> Add1/1
  Product2/1 -> Add1/2
  Alpha1/1 -> Produc3t/1
  Sin_Coefficient1/1 -> Produc3t/2
  Cos_Coefficient1/1 -> Product4/2
  Beta1/1 -> Product4/1
  Alpha/1 -> Product1/1
  Cos_Coefficient/1 -> Product1/2
  Beta/1 -> Product2/1
  Sin_Coefficient/1 -> Product2/2
  Add1/1 -> D/1
  Add2/1 -> Q/1

== system FOC_Motor_Control/Motor_Control/Motor_Control_Function/FOC_Control_100us/FOC/Q_Current_PI ==
  Reset : Inport
  Bus_voltage : Inport  Port=2
  Current_Command : Inport  Port=3
  Current_Measured : Inport  Port=4
  Add2 : Sum  Inputs=|+-
  IQ_Control : Subsystem
  Vq_voltage : Outport  VectorParamsAs1DForOutWhenUnconnected=off
  wires:
  Current_Command/1 -> Add2/1
  Current_Measured/1 -> Add2/2
  Add2/1 -> IQ_Control/3(Err)  "currentControlError"
  Reset/1 -> IQ_Control/1(Reset)
  Bus_voltage/1 -> IQ_Control/2(Bus_voltage)
  IQ_Control/1(PI_Out) -> Vq_voltage/1

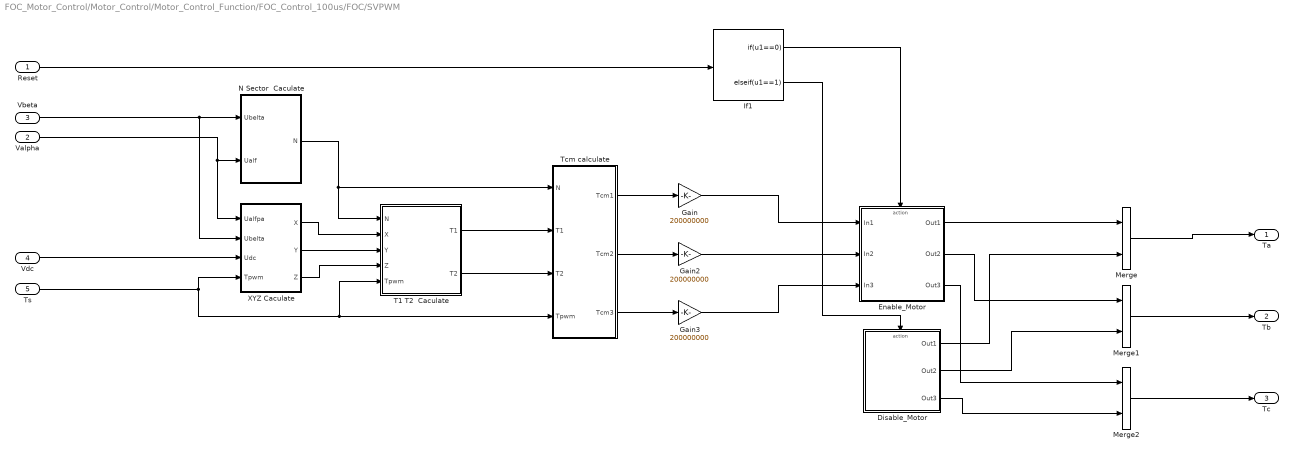
== system FOC_Motor_Control/Motor_Control/Motor_Control_Function/FOC_Control_100us/FOC/SVPWM ==
  Reset : Inport
  Valpha : Inport  Port=2
  Vbeta : Inport  Port=3
  Vdc : Inport  Port=4
  Ts : Inport  Port=5
  Disable_Motor : Subsystem  TreatAsAtomicUnit=on
  Enable_Motor : Subsystem  TreatAsAtomicUnit=on
  Gain : Gain  Gain=200000000
  Gain2 : Gain  Gain=200000000
  Gain3 : Gain  Gain=200000000
  If1 : If  IfExpression=u1==0  ElseIfExpressions=u1==1  ShowElse=off
  Merge : Merge
  Merge1 : Merge
  Merge2 : Merge
  N Sector  Caculate : Subsystem  TreatAsAtomicUnit=on
  T1 T2  Caculate : Subsystem  TreatAsAtomicUnit=on
  Tcm calculate : Subsystem  TreatAsAtomicUnit=on
  XYZ Caculate : Subsystem  TreatAsAtomicUnit=on
  Ta : Outport
  Tb : Outport  Port=2
  Tc : Outport  Port=3
  wires:
  T1 T2  Caculate/2(T2) -> Tcm calculate/3(T2)
  XYZ Caculate/1(X) -> T1 T2  Caculate/2(X)
  N Sector  Caculate/1(N) -> T1 T2  Caculate/1(N), Tcm calculate/1(N)
  Vdc/1 -> XYZ Caculate/3(Udc)
  T1 T2  Caculate/1(T1) -> Tcm calculate/2(T1)
  XYZ Caculate/3(Z) -> T1 T2  Caculate/4(Z)
  XYZ Caculate/2(Y) -> T1 T2  Caculate/3(Y)
  Valpha/1 -> N Sector  Caculate/2(Ualf), XYZ Caculate/1(Ualfpa)
  Vbeta/1 -> N Sector  Caculate/1(Ubelta), XYZ Caculate/2(Ubelta)
  Ts/1 -> T1 T2  Caculate/5(Tpwm), Tcm calculate/4(Tpwm), XYZ Caculate/4(Tpwm)
  Gain/1 -> Enable_Motor/1(In1)
  Gain2/1 -> Enable_Motor/2(In2)
  Reset/1 -> If1/1
  If1/1 -> Enable_Motor/Action
  If1/2 -> Disable_Motor/Action
  Gain3/1 -> Enable_Motor/3(In3)
  Enable_Motor/1(Out1) -> Merge/1
  Disable_Motor/1(Out1) -> Merge/2
  Enable_Motor/2(Out2) -> Merge1/1
  Disable_Motor/2(Out2) -> Merge1/2
  Enable_Motor/3(Out3) -> Merge2/1
  Disable_Motor/3(Out3) -> Merge2/2
  Merge/1 -> Ta/1
  Merge1/1 -> Tb/1
  Merge2/1 -> Tc/1
  Tcm calculate/1(Tcm1) -> Gain/1
  Tcm calculate/2(Tcm2) -> Gain2/1
  Tcm calculate/3(Tcm3) -> Gain3/1

== system FOC_Motor_Control/Motor_Control/Motor_Control_Function/FOC_Control_100us/FOC/Sine_Cosine ==
  note: Sine Cosine Coefficients
  P : Inport
  Cosine : Lookup_n-D  NumberOfTableDimensions=1  LookupTableObject=''  BreakpointsForDimension1=[0:2*pi/4095:2*pi]  BreakpointsForDimension1FirstPoint=10  BreakpointsForDimension2FirstPoint=10  BreakpointsForDimension1Spacing=12  BreakpointsForDimension2Spacing=12  IndexSearchMethod=Evenly spaced points  Table=Cosine_table  InterpMethod=Flat  DiagnosticForOutOfRangeInput=Error  InternalRulePriority=Speed  RndMeth=Simplest  InputSameDT=on
  Saturation : Saturate  UpperLimit=2*pi-0.0001  LowerLimit=0+0.0001
  Scope : Scope  NumInputPorts=2
  Sine : Lookup_n-D  NumberOfTableDimensions=1  LookupTableObject=''  BreakpointsForDimension1=[0:2*pi/4095:2*pi]  BreakpointsForDimension1FirstPoint=10  BreakpointsForDimension2FirstPoint=10  BreakpointsForDimension1Spacing=12  BreakpointsForDimension2Spacing=12  IndexSearchMethod=Evenly spaced points  Table=Sine_table  InterpMethod=Flat  DiagnosticForOutOfRangeInput=Error  InternalRulePriority=Speed  RndMeth=Simplest  InputSameDT=on
  Sin : Outport  VectorParamsAs1DForOutWhenUnconnected=off
  Cos : Outport  Port=2  VectorParamsAs1DForOutWhenUnconnected=off
  wires:
  P/1 -> Saturation/1  "position"
  Sine/1 -> Scope/1, Sin/1
  Cosine/1 -> Scope/2, Cos/1
  Saturation/1 -> Cosine/1, Sine/1

== system FOC_Motor_Control/Motor_Control/Motor_Control_Function/Angle_Speed_100us/Speed_Resolver/Speed_cacl/LPF ==
  u : Inport
  Add : Sum  Inputs=+-
  Add1 : Sum
  Constant1 : Constant  Value=SpeedFilter_Fn  OutDataTypeStr=single
  Divide1 : Product  Inputs=**
  Unit Delay : UnitDelay  SampleTime=-1  HasFrameUpgradeWarning=on
  y : Outport
  wires:
  Constant1/1 -> Divide1/1
  u/1 -> Add/1
  Add/1 -> Divide1/2
  Divide1/1 -> Add1/1
  Unit Delay/1 -> Add/2, Add1/2
  Add1/1 -> Unit Delay/1, y/1

== system FOC_Motor_Control/Motor_Control/Motor_Control_Function/Control_Command_2ms/Control_Command_2ms/Speed_PI/SpeedLoop ==
  CMD_RPM : Inport  OutDataTypeStr=single
  FdkRPM : Inport  Port=2  OutDataTypeStr=single
  Reset : Inport  Port=3
  Constant : Constant  Value=LADRC_b0  OutDataTypeStr=single  SampleTime=-1
  Divide : Product  Inputs=*/  OutDataTypeStr=single
  LESO : Subsystem
  Saturation : Saturate  UpperLimit=Speed_PI_OutputMax  LowerLimit=Speed_PI_OutputMin  OutDataTypeStr=single
  Sum : Sum  Inputs=|+-  OutDataTypeStr=single
  Sum1 : Sum  Inputs=|+-  OutDataTypeStr=single
  Unit Delay : UnitDelay  SampleTime=-1  HasFrameUpgradeWarning=on
  omega_c : Gain  Gain=LADRC_Omega_c  OutDataTypeStr=single
  RefIq : Outport  OutDataTypeStr=single
  wires:
  Saturation/1 -> RefIq/1, Unit Delay/1
  Constant/1 -> Divide/2
  Divide/1 -> Saturation/1
  LESO/2(f_hat) -> Sum1/2
  FdkRPM/1 -> LESO/1(FbkSpd)  "FdkRPM"
  LESO/1(omega_r_hat) -> Sum/2
  Sum1/1 -> Divide/1
  omega_c/1 -> Sum1/1
  Sum/1 -> omega_c/1
  CMD_RPM/1 -> Sum/1  "CMD_RPM"
  Unit Delay/1 -> LESO/2(iq)
  Reset/1 -> LESO/3(Reset)

== system FOC_Motor_Control/Motor_Control/Motor_Control_Function/Control_Command_2ms/Control_Command_2ms/Speed_PI/Speed_PI ==
  Ref : Inport
  Fdk : Inport  Port=2
  Reset : Inport  Port=3
  Speed_Control : Subsystem
  Sum : Sum  Inputs=|+-
  PI_out : Outport  VectorParamsAs1DForOutWhenUnconnected=off
  wires:
  Speed_Control/1(PI_Out) -> PI_out/1
  Reset/1 -> Speed_Control/2(Reset)
  Ref/1 -> Sum/1
  Sum/1 -> Speed_Control/1(Err)
  Fdk/1 -> Sum/2

== system FOC_Motor_Control/Motor_Control/Motor_Control_Function/FOC_Control_100us/FOC/Clarke_Transform/Clark1 ==
  Iabc : Inport
  Add : Sum  Inputs=+--
  Add1 : Sum  Inputs=+-
  Demux : Demux  Outputs=3
  Gain : Gain  Gain=0.5
  Gain1 : Gain  Gain=0.5
  Gain2 : Gain  Gain=sqrt(2/3)
  Gain3 : Gain  Gain=sqrt(3)/2
  Gain4 : Gain  Gain=sqrt(3)/2
  Gain5 : Gain  Gain=sqrt(2/3)
  Ialpha : Outport  VectorParamsAs1DForOutWhenUnconnected=off
  Ibeta : Outport  Port=2  VectorParamsAs1DForOutWhenUnconnected=off
  wires:
  Iabc/1 -> Demux/1
  Demux/1 -> Add/1
  Gain/1 -> Add/2
  Demux/2 -> Gain3/1, Gain/1
  Gain1/1 -> Add/3
  Demux/3 -> Gain4/1, Gain1/1
  Add/1 -> Gain2/1
  Gain2/1 -> Ialpha/1
  Gain3/1 -> Add1/1
  Gain4/1 -> Add1/2
  Add1/1 -> Gain5/1
  Gain5/1 -> Ibeta/1

== system FOC_Motor_Control/Motor_Control/Motor_Control_Function/FOC_Control_100us/FOC/DT_Compensation/DT_Compensation ==
  Ts : Inport
  Td : Inport  Port=2
  Udc : Inport  Port=3
  Id : Inport  Port=4
  Iq : Inport  Port=5
  Theta : Inport  Port=6
  Enable : EnablePort
  Fcn : Fcn  Expr=u(1)*u(3)/u(2)
  IsTheta_Cal : Subsystem
  Mux : Mux  Inputs=3
  Scope : Scope
  Subsystem : Subsystem
  Uabc_alphabeta : Subsystem
  Delta_Ualpha : Outport
  Delta_Ubeta : Outport  Port=2
  wires:
  Udc/1 -> Mux/3
  Ts/1 -> Mux/2
  Td/1 -> Mux/1
  Mux/1 -> Fcn/1
  Fcn/1 -> Subsystem/1(Err_Voltage)
  Id/1 -> IsTheta_Cal/1(Id)
  Iq/1 -> IsTheta_Cal/2(Iq)
  Theta/1 -> IsTheta_Cal/3(d_theta)
  IsTheta_Cal/1(IsTheta) -> Scope/1, Subsystem/2(Istheta)
  Subsystem/1(Uabcc) -> Uabc_alphabeta/1(Uabc)
  Uabc_alphabeta/1(Ualpha) -> Delta_Ualpha/1
  Uabc_alphabeta/2(Ubeta) -> Delta_Ubeta/1

== system FOC_Motor_Control/Motor_Control/Motor_Control_Function/FOC_Control_100us/FOC/D_Current_PI/ID_Control ==
  Reset : Inport
  Bus_voltage : Inport  Port=2
  Err : Inport  Port=3
  Add : Sum
  Cons : Constant  Value=0  OutDataTypeStr=single
  Discrete-Time Integrator : DiscreteIntegrator  ExternalReset=level  SampleTime=-1  ICPrevOutput=DiscIntNeverNeededParam  ICPrevScaledInput=DiscIntNeverNeededParam
  Ki : Constant  Value=ID_Ki  OutDataTypeStr=single
  Kp : Constant  Value=ID_Kp  OutDataTypeStr=single
  Normal : Subsystem  TreatAsAtomicUnit=on
  Product : Product
  Product1 : Product
  Relational Operator1 : RelationalOperator  Operator===  OutDataTypeStr=boolean  RndMeth=Simplest
  Saturation Dynamic : simulink/Discontinuities/Saturation Dynamic  OutMin=[]  OutMax=[]  OutDataTypeStr=Inherit: Same as second input  OutDataType=fixdt(1, 16)  OutScaling=2^-10  DoSatur=off
  Switch : Switch  Criteria=u2 > Threshold
  Unit Delay3 : UnitDelay  SampleTime=-1  HasFrameUpgradeWarning=on
  PI_Out : Outport
  wires:
  Kp/1 -> Product/1
  Err/1 -> Product/2, Switch/1
  Switch/1 -> Product1/2
  Product1/1 -> Discrete-Time Integrator/1
  Product/1 -> Add/1
  Add/1 -> Saturation Dynamic/2, Relational Operator1/1
  Saturation Dynamic/1 -> Relational Operator1/2, PI_Out/1
  Cons/1 -> Switch/3
  Discrete-Time Integrator/1 -> Add/2
  Relational Operator1/1 -> Unit Delay3/1
  Ki/1 -> Product1/1
  Unit Delay3/1 -> Switch/2
  Reset/1 -> Discrete-Time Integrator/2
  Bus_voltage/1 -> Normal/1(Bus_voltage)
  Normal/1(Out1) -> Saturation Dynamic/1
  Normal/2(Out2) -> Saturation Dynamic/3

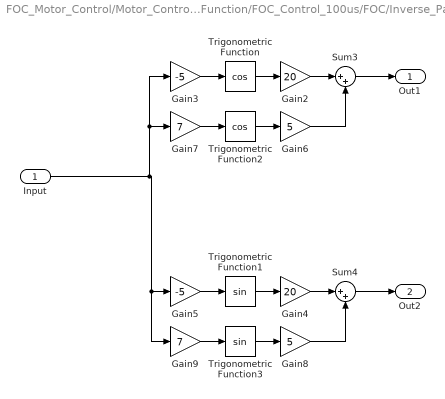
== system FOC_Motor_Control/Motor_Control/Motor_Control_Function/FOC_Control_100us/FOC/Inverse_Park_Transform/Harmonic_injection ==
  Input : Inport
  Gain2 : Gain  Gain=20
  Gain3 : Gain  Gain=-5
  Gain4 : Gain  Gain=20
  Gain5 : Gain  Gain=-5
  Gain6 : Gain  Gain=5
  Gain7 : Gain  Gain=7
  Gain8 : Gain  Gain=5
  Gain9 : Gain  Gain=7
  Sum3 : Sum  Inputs=|++
  Sum4 : Sum  Inputs=|++
  Trigonometric Function : Trigonometry  Operator=cos
  Trigonometric Function1 : Trigonometry
  Trigonometric Function2 : Trigonometry  Operator=cos
  Trigonometric Function3 : Trigonometry
  Out1 : Outport
  Out2 : Outport  Port=2
  wires:
  Trigonometric Function1/1 -> Gain4/1
  Trigonometric Function/1 -> Gain2/1
  Gain5/1 -> Trigonometric Function1/1
  Trigonometric Function2/1 -> Gain6/1
  Gain7/1 -> Trigonometric Function2/1
  Gain9/1 -> Trigonometric Function3/1
  Trigonometric Function3/1 -> Gain8/1
  Gain2/1 -> Sum3/1
  Gain3/1 -> Trigonometric Function/1
  Gain4/1 -> Sum4/1
  Gain6/1 -> Sum3/2
  Gain8/1 -> Sum4/2
  Sum3/1 -> Out1/1
  Sum4/1 -> Out2/1
  Input/1 -> Gain9/1, Gain5/1, Gain3/1, Gain7/1

== system FOC_Motor_Control/Motor_Control/Motor_Control_Function/FOC_Control_100us/FOC/Q_Current_PI/IQ_Control ==
  Reset : Inport
  Bus_voltage : Inport  Port=2
  Err : Inport  Port=3
  Add : Sum
  Cons : Constant  Value=0  OutDataTypeStr=single
  Discrete-Time Integrator : DiscreteIntegrator  ExternalReset=level  SampleTime=-1  ICPrevOutput=DiscIntNeverNeededParam  ICPrevScaledInput=DiscIntNeverNeededParam
  Ki : Constant  Value=IQ_Ki  OutDataTypeStr=single
  Kp : Constant  Value=IQ_Kp  OutDataTypeStr=single
  Normal : Subsystem  TreatAsAtomicUnit=on
  Product : Product
  Product1 : Product
  Relational Operator1 : RelationalOperator  Operator===  OutDataTypeStr=boolean  RndMeth=Simplest
  Saturation Dynamic : simulink/Discontinuities/Saturation Dynamic  OutMin=[]  OutMax=[]  OutDataTypeStr=Inherit: Same as second input  OutDataType=fixdt(1, 16)  OutScaling=2^-10  DoSatur=off
  Switch : Switch  Criteria=u2 > Threshold
  Unit Delay3 : UnitDelay  SampleTime=-1  HasFrameUpgradeWarning=on
  PI_Out : Outport
  wires:
  Kp/1 -> Product/1
  Err/1 -> Switch/1, Product/2
  Switch/1 -> Product1/2
  Product1/1 -> Discrete-Time Integrator/1
  Product/1 -> Add/1
  Add/1 -> Saturation Dynamic/2, Relational Operator1/1
  Saturation Dynamic/1 -> PI_Out/1, Relational Operator1/2
  Cons/1 -> Switch/3
  Discrete-Time Integrator/1 -> Add/2
  Relational Operator1/1 -> Unit Delay3/1
  Ki/1 -> Product1/1
  Unit Delay3/1 -> Switch/2
  Reset/1 -> Discrete-Time Integrator/2
  Bus_voltage/1 -> Normal/1(Bus_voltage)
  Normal/1(Out1) -> Saturation Dynamic/1
  Normal/2(Out2) -> Saturation Dynamic/3

== system FOC_Motor_Control/Motor_Control/Motor_Control_Function/FOC_Control_100us/FOC/SVPWM/Disable_Motor ==
  Action Port : ActionPort  ActionPortLabel=elseif(u1==1)
  Constant : Constant  Value=0  OutDataTypeStr=single
  Constant1 : Constant  Value=0  OutDataTypeStr=single
  Constant2 : Constant  Value=0  OutDataTypeStr=single
  Out1 : Outport
  Out2 : Outport  Port=2
  Out3 : Outport  Port=3
  wires:
  Constant/1 -> Out1/1
  Constant1/1 -> Out2/1
  Constant2/1 -> Out3/1

== system FOC_Motor_Control/Motor_Control/Motor_Control_Function/FOC_Control_100us/FOC/SVPWM/Enable_Motor ==
  In1 : Inport
  In2 : Inport  Port=2
  In3 : Inport  Port=3
  Action Port : ActionPort  ActionPortLabel=if(u1==0)
  Out1 : Outport
  Out2 : Outport  Port=2
  Out3 : Outport  Port=3
  wires:
  In1/1 -> Out1/1
  In2/1 -> Out2/1
  In3/1 -> Out3/1

== system FOC_Motor_Control/Motor_Control/Motor_Control_Function/FOC_Control_100us/FOC/SVPWM/N Sector  Caculate ==
  Ubelta : Inport
  Ualf : Inport  Port=2
  Add : Sum  Inputs=+++
  Add1 : Sum  Inputs=-+
  Add2 : Sum  Inputs=--
  Constant : Constant  OutDataTypeStr=single
  Constant1 : Constant  Value=0  OutDataTypeStr=single
  Gain : Gain  Gain=sqrt(3)
  Gain1 : Gain  Gain=2
  Gain2 : Gain  Gain=4
  Saturation : Saturate  UpperLimit=6  LowerLimit=1
  Switch : Switch
  Switch1 : Switch
  Switch2 : Switch
  N : Outport
  wires:
  Saturation/1 -> N/1
  Add/1 -> Saturation/1
  Gain2/1 -> Add/3
  Switch2/1 -> Gain2/1
  Add2/1 -> Switch2/2
  Gain1/1 -> Add/2
  Switch1/1 -> Gain1/1
  Add1/1 -> Switch1/2
  Gain/1 -> Add2/2, Add1/2
  Ualf/1 -> Gain/1
  Switch/1 -> Add/1
  Constant1/1 -> Switch/3, Switch1/3, Switch2/3
  Constant/1 -> Switch/1, Switch1/1, Switch2/1
  Ubelta/1 -> Add2/1, Add1/1, Switch/2

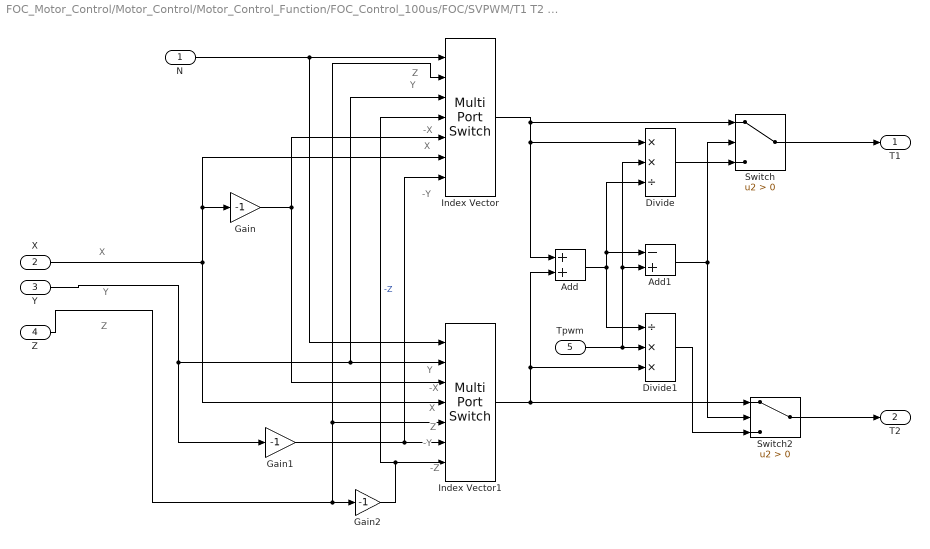
== system FOC_Motor_Control/Motor_Control/Motor_Control_Function/FOC_Control_100us/FOC/SVPWM/T1 T2  Caculate ==
  note: Z
  note: Y
  note: -X
  note: X
  note: -Y
  note: Y
  note: -X
  note: X
  note: Z
  note: -Y
  note: -Z
  note: X
  note: Y
  note: Z
  N : Inport
  X : Inport  Port=2
  Y : Inport  Port=3
  Z : Inport  Port=4
  Tpwm : Inport  Port=5
  Add : Sum
  Add1 : Sum  Inputs=-+
  Divide : Product  Inputs=**/
  Divide1 : Product  Inputs=/**
  Gain : Gain  Gain=-1
  Gain1 : Gain  Gain=-1
  Gain2 : Gain  Gain=-1
  Index Vector : MultiPortSwitch  Inputs=6
  Index Vector1 : MultiPortSwitch  Inputs=6
  Switch : Switch  Criteria=u2 > Threshold
  Switch2 : Switch  Criteria=u2 > Threshold
  T1 : Outport
  T2 : Outport  Port=2
  wires:
  Switch2/1 -> T2/1
  Divide1/1 -> Switch2/3
  Switch/1 -> T1/1
  Add1/1 -> Switch/2, Switch2/2
  Add/1 -> Divide1/1, Divide/3, Add1/1
  Tpwm/1 -> Divide1/2, Divide/2, Add1/2
  Divide/1 -> Switch/3
  Index Vector1/1 -> Switch2/1, Add/2, Divide1/3
  Index Vector/1 -> Switch/1, Divide/1, Add/1
  Gain1/1 -> Index Vector/7, Index Vector1/6
  Gain2/1 -> Index Vector/4, Index Vector1/7  "-Z"
  Gain/1 -> Index Vector/5, Index Vector1/3
  Y/1 -> Gain1/1, Index Vector/3, Index Vector1/2
  X/1 -> Index Vector1/4, Index Vector/6, Gain/1
  Z/1 -> Index Vector/2, Index Vector1/5, Gain2/1
  N/1 -> Index Vector1/1, Index Vector/1

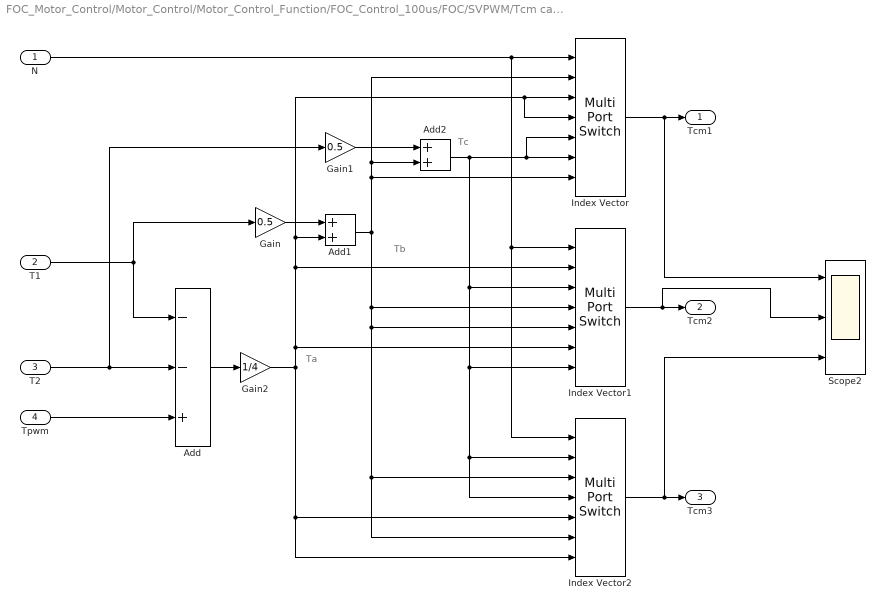
== system FOC_Motor_Control/Motor_Control/Motor_Control_Function/FOC_Control_100us/FOC/SVPWM/Tcm calculate ==
  note: Tc
  note: Tb
  note: Ta
  N : Inport
  T1 : Inport  Port=2
  T2 : Inport  Port=3
  Tpwm : Inport  Port=4
  Add : Sum  Inputs=--+
  Add1 : Sum
  Add2 : Sum
  Gain : Gain  Gain=0.5
  Gain1 : Gain  Gain=0.5
  Gain2 : Gain  Gain=1/4
  Index Vector : MultiPortSwitch  Inputs=6
  Index Vector1 : MultiPortSwitch  Inputs=6
  Index Vector2 : MultiPortSwitch  Inputs=6
  Scope2 : Scope  NumInputPorts=3
  Tcm1 : Outport
  Tcm2 : Outport  Port=2
  Tcm3 : Outport  Port=3
  wires:
  Index Vector2/1 -> Scope2/3, Tcm3/1
  N/1 -> Index Vector/1, Index Vector1/1, Index Vector2/1
  Add2/1 -> Index Vector/5, Index Vector/6, Index Vector1/3, Index Vector1/7, Index Vector2/2, Index Vector2/4
  Gain1/1 -> Add2/1
  Add1/1 -> Add2/2, Index Vector/2, Index Vector/7, Index Vector1/4, Index Vector1/5, Index Vector2/3, Index Vector2/6
  Gain2/1 -> Index Vector2/5, Index Vector2/7, Add1/2, Index Vector/3, Index Vector/4, Index Vector1/2, Index Vector1/6
  Gain/1 -> Add1/1
  Add/1 -> Gain2/1
  Tpwm/1 -> Add/3
  T2/1 -> Add/2, Gain1/1
  T1/1 -> Add/1, Gain/1
  Index Vector/1 -> Scope2/1, Tcm1/1
  Index Vector1/1 -> Scope2/2, Tcm2/1
